simulink model "pulse_detector_v1_1"  (R2017b)
settings: Solver=VariableStepAuto  StartTime=0.0  StopTime=SimTime  RelTol=1e-3
undefined symbols (not defined in the file): CorrFilter, threshold, WindowLen
libraries: simulink x1, dspsrcs4 x1, hdlsllib x1
settings Model: SimulationMode=accelerator  Creator=proso  LastModifiedBy=proso
settings DataIOCC: ReturnWorkspaceOutputs=on

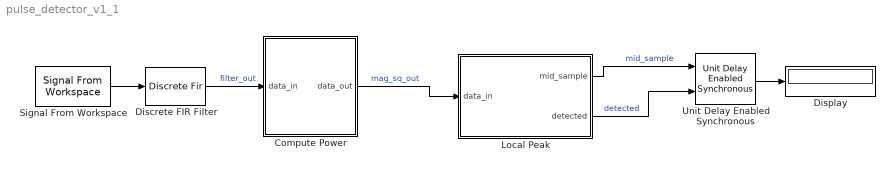
== system pulse_detector_v1_1 ==
  Compute Power : Subsystem
  Discrete FIR Filter : DiscreteFir  Coefficients=CorrFilter
  Display : Display
  Local Peak : Subsystem
  Signal From Workspace : dspsrcs4/Signal From Workspace  X=RxSignal  Ts=1  nsamps=1  OutputAfterFinalValue=Setting to zero  ignoreOrWarnInputAndFrameLengths=off  OutputFrames=off
  Unit Delay Enabled Synchronous : hdlsllib/Discrete/Unit Delay Enabled Synchronous  InitialCondition=0.0  SampleTime=-1
      settings: SourceProductName=HDL Coder  SourceProductBaseCode=HD
  wires:
  Signal From Workspace/1 -> Discrete FIR Filter/1
  Discrete FIR Filter/1 -> Compute Power/1(data_in)  "filter_out"
  Unit Delay Enabled Synchronous/1 -> Display/1
  Compute Power/1(data_out) -> Local Peak/1(data_in)  "mag_sq_out"
  Local Peak/1(mid_sample) -> Unit Delay Enabled Synchronous/1  "mid_sample"
  Local Peak/2(detected) -> Unit Delay Enabled Synchronous/2  "detected"

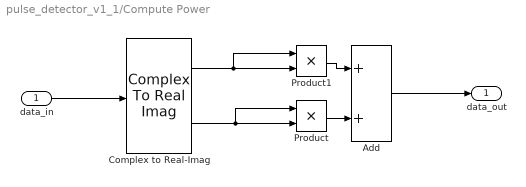
== system pulse_detector_v1_1/Compute Power ==
  data_in : Inport
  Add : Sum
  Complex to Real-Imag : ComplexToRealImag
  Product : Product
  Product1 : Product
  data_out : Outport
  wires:
  Product1/1 -> Add/1
  data_in/1 -> Complex to Real-Imag/1
  Complex to Real-Imag/1 -> Product1/1, Product1/2
  Add/1 -> data_out/1
  Product/1 -> Add/2
  Complex to Real-Imag/2 -> Product/1, Product/2

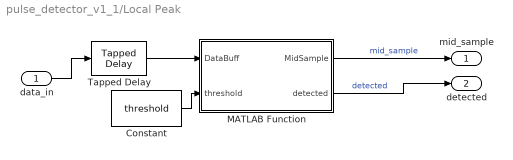
== system pulse_detector_v1_1/Local Peak ==
  data_in : Inport
  Constant : Constant  Value=threshold
  MATLAB Function : MATLAB Function  TreatAsAtomicUnit=on
  Tapped Delay : simulink/Discrete/Tapped Delay  vinit=0.0  samptime=-1  NumDelays=WindowLen  DelayOrder=Oldest  includeCurrent=off
  mid_sample : Outport
  detected : Outport  Port=2
  wires:
  MATLAB Function/1(MidSample) -> mid_sample/1  "mid_sample"
  data_in/1 -> Tapped Delay/1
  Constant/1 -> MATLAB Function/2(threshold)
  MATLAB Function/2(detected) -> detected/1  "detected"
  Tapped Delay/1 -> MATLAB Function/1(DataBuff)

== matlab function pulse_detector_v1_1/Local Peak/MATLAB Function ==
  data: MidSample output; DataBuff input; threshold input; detected output; WindowLen parameter
function [MidSample,detected] = fcn(DataBuff,threshold, WindowLen)
   
MidIdx = ceil(WindowLen/2);
% Sliding window operation

% Compare each value in the window to the middle sample via subtraction
MidSample = DataBuff(MidIdx);
CompareOut = DataBuff - MidSample; % this is a vector

% if all values in the result are negative and the middle sample is
% greater than a threshold, it is a local max
if all(CompareOut <= 0) && (MidSample > threshold)
    detected =1;
else 
    detected = 0;
end
